simulink model "equalizer"  (Simulink 5.0)
settings: Solver=ode45  StartTime=0.0  StopTime=1  RelTol=1e-3
libraries: dspsigops x10, dsparch4 x2, commsink2 x2, commrandsrc2 x1
settings Model: LastModifiedBy=Daiming Qu  RTWOptions="-aEnforceIntegerDowncast=1 -aExtMode=0 -aExtModeTesting=0 -aFoldNonRolledExpr=1 -aForceParamTrailComments=0 -aGenerateComments=1 -aGenerateReport=0 -aIgnoreCustomStorageClasses=1 -aIncDataTypeInIds=0 -aIncHierarchyInIds=0 -aInlineInvariantSignals=0 -aInlinedPrmAccess=\"Literals\" -aLocalBlockOutputs=1 -aLogVarNameModifier=\"rt_\" -aMaxRTWIdLen=31 -aPrefixModelToSubsysFcnNames=1 -aRTWVerbose=1 -aRollThreshold=5 -aShowEliminatedStatements=0"

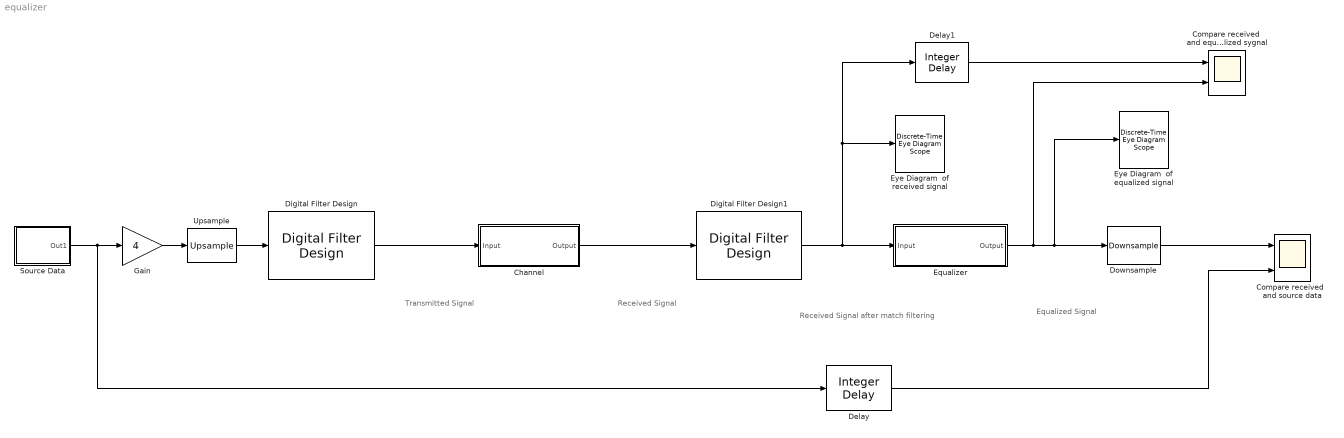
== system equalizer ==
  note: Transmitted Signal
  note: Received Signal
  note: Equalized Signal
  note: Received Signal
      | after match filtering
  " Delay" : dspsigops/Integer Delay  delay=11  ic=0  reset_popup=None
  Channel : Subsystem  Tag=FilterWizardSubSystem
  Compare received  and equalized sygnal : Scope  NumInputPorts=2
      settings: YMin=-5~-5  YMax=5~5  SaveName=ScopeData2
  Compare received   and source data : Scope  NumInputPorts=2
      settings: YMin=-2~-2  YMax=2~2
  Delay1 : dspsigops/Integer Delay  delay=4  ic=0  reset_popup=None
  Digital Filter Design : dsparch4/Digital Filter Design
  Digital Filter Design1 : dsparch4/Digital Filter Design
  Downsample : dspsigops/Downsample  N=4  phase=0  ic=0  smode=Allow multirate  fmode=Maintain input frame size
  Equalizer : Subsystem  Tag=FilterWizardSubSystem  Description=equalizer
  Eye Diagram  of equalized signal : commsink2/Discrete-Time Eye Diagram Scope  Tag=EyeDiagram  showPlotting=off  sampPerSymb=8  offsetEye=0  symbPerTrace=1  numTraces=40  numNewFrames=10  showRendering=off  LineMarkers=None  LineStyles=-  LineColors=[0 0 0]  dupPoints=on  fading=on  render=on  AxisGrid=on  showAxes=on  yMin=-2  yMax=2  inphaseLabel=In-phase Amplitude  quadratureLabel=Quadrature Amplitude  showFigure=on  openScopeAtSimStart=on  dispDiagram=In-phase Only  FrameNumber=off  FigPos=[412 42 560 487]  figTitle=Eye Diagram  block_type_=eye  numLinesMax=8
  Eye Diagram  of received signal : commsink2/Discrete-Time Eye Diagram Scope  Tag=EyeDiagram  showPlotting=off  sampPerSymb=8  offsetEye=0  symbPerTrace=1  numTraces=40  numNewFrames=10  showRendering=off  LineStyles=-  LineColors=[0 0 0]  dupPoints=on  fading=on  render=on  AxisGrid=on  showAxes=on  yMin=-2  yMax=2  inphaseLabel=In-phase Amplitude  quadratureLabel=Quadrature Amplitude  showFigure=on  openScopeAtSimStart=on  dispDiagram=In-phase Only  FrameNumber=off  FigPos=[10 42 560 487]  figTitle=Eye Diagram  block_type_=eye  numLinesMax=8
  Gain : Gain  Gain=4  SaturateOnIntegerOverflow=on
  Source Data : Subsystem
  Upsample : dspsigops/Upsample  N=4  phase=0  ic=0  mode=Maintain input frame size
  wires:
  Source Data/1(Out1) -> " Delay"/1, Gain/1
  Upsample/1 -> Digital Filter Design/1
  Equalizer/1(Output) -> Eye Diagram  of equalized signal/1, Downsample/1, Compare received  and equalized sygnal/2
  Downsample/1 -> Compare received   and source data/1
  " Delay"/1 -> Compare received   and source data/2
  Digital Filter Design/1 -> Channel/1(Input)
  Digital Filter Design1/1 -> Equalizer/1(Input), Eye Diagram  of received signal/1, Delay1/1
  Channel/1(Output) -> Digital Filter Design1/1
  Delay1/1 -> Compare received  and equalized sygnal/1
  Gain/1 -> Upsample/1

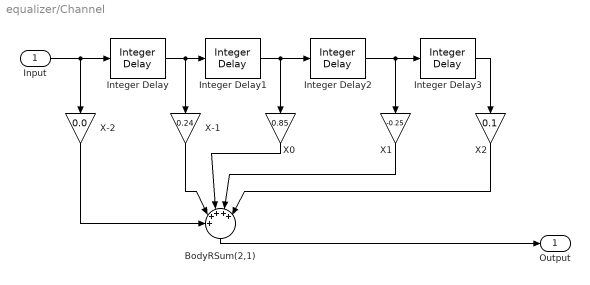
== system equalizer/Channel ==
  Input : Inport
  BodyRSum(2,1) : Sum  Orientation=down  Inputs=+++++|  SaturateOnIntegerOverflow=on  InputSameDT=on
  Integer Delay{,1..3} (4 alike) : dspsigops/Integer Delay  delay=4  ic=0  reset_popup=None
  X-1 : Gain  Orientation=down  Gain=0.24  SaturateOnIntegerOverflow=on
  X-2 : Gain  Orientation=down  Gain=0.0  SaturateOnIntegerOverflow=on
  X0 : Gain  Orientation=down  Gain=0.85  SaturateOnIntegerOverflow=on
  X1 : Gain  Orientation=down  Gain=-0.25  SaturateOnIntegerOverflow=on
  X2 : Gain  Orientation=down  Gain=0.1  SaturateOnIntegerOverflow=on
  Output : Outport
  wires:
  Input/1 -> X-2/1, Integer Delay/1
  Integer Delay/1 -> X-1/1, Integer Delay1/1
  X-2/1 -> BodyRSum(2,1)/1
  X-1/1 -> BodyRSum(2,1)/2
  Integer Delay1/1 -> X0/1, Integer Delay2/1
  X0/1 -> BodyRSum(2,1)/3
  BodyRSum(2,1)/1 -> Output/1
  Integer Delay2/1 -> X1/1, Integer Delay3/1
  X1/1 -> BodyRSum(2,1)/4
  X2/1 -> BodyRSum(2,1)/5
  Integer Delay3/1 -> X2/1

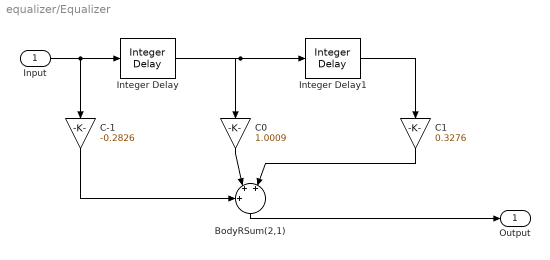
== system equalizer/Equalizer ==
  Input : Inport
  BodyRSum(2,1) : Sum  Orientation=down  Inputs=+++|  SaturateOnIntegerOverflow=on  InputSameDT=on
  C-1 : Gain  Orientation=down  Gain=-0.2826  SaturateOnIntegerOverflow=on
  C0 : Gain  Orientation=down  Gain=1.0009  SaturateOnIntegerOverflow=on
  C1 : Gain  Orientation=down  Gain=0.3276  SaturateOnIntegerOverflow=on
  Integer Delay : dspsigops/Integer Delay  delay=4  ic=0  reset_popup=None
  Integer Delay1 : dspsigops/Integer Delay  delay=4  ic=0  reset_popup=None
  Output : Outport
  wires:
  Input/1 -> C-1/1, Integer Delay/1
  Integer Delay/1 -> C0/1, Integer Delay1/1
  C-1/1 -> BodyRSum(2,1)/1
  C0/1 -> BodyRSum(2,1)/2
  Integer Delay1/1 -> C1/1
  C1/1 -> BodyRSum(2,1)/3
  BodyRSum(2,1)/1 -> Output/1

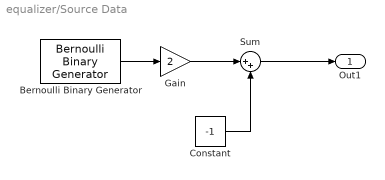
== system equalizer/Source Data ==
  Bernoulli Binary Generator : commrandsrc2/Bernoulli Binary Generator  P=0.5  seed=34  Ts=0.001  frameBased=off  sampPerFrame=1  orient=off
  Constant : Constant  Value=-1
  Gain : Gain  Gain=2  SaturateOnIntegerOverflow=on
  Sum : Sum  Inputs=|++  SaturateOnIntegerOverflow=on
  Out1 : Outport
  wires:
  Bernoulli Binary Generator/1 -> Gain/1
  Gain/1 -> Sum/1
  Sum/1 -> Out1/1
  Constant/1 -> Sum/2
